simulink model "FoilSimulation23a"  (R2023a)
settings: Solver=VariableStepAuto  StartTime=0.0  StopTime=TF  RelTol=1e-3
values from neighbouring files (symbols this model uses):
  U = 0    [init.m]
  x0 = [5 ... (first row only)    [init.m]
undefined symbols (not defined in the file or in its folder): hydrofoil_model
settings Model: Creator=alank  LastModifiedBy=alank
settings RTWCC: GPUComputeCapability=5.0

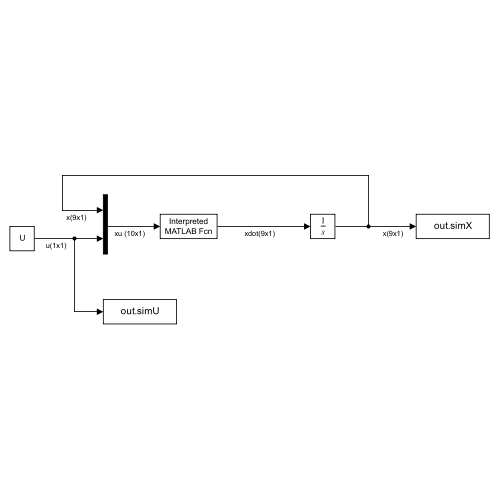
[thumbnail: Simulink's stored preview of the top-level diagram]
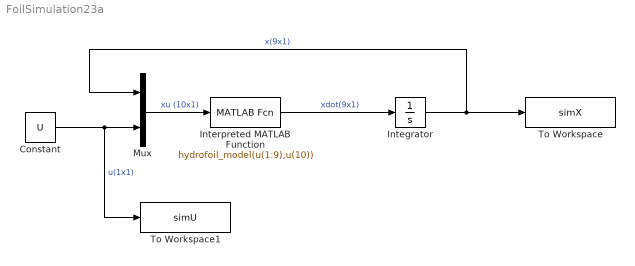
== system FoilSimulation23a ==
  Constant : Constant  Value=U
  Integrator : Integrator  InitialCondition=x0
  Interpreted MATLAB Function : MATLABFcn  MATLABFcn=hydrofoil_model(u(1:9),u(10))
  Mux : Mux  Inputs=2
  To Workspace : ToWorkspace  VariableName=simX  SaveFormat=Timeseries  SampleTime=-1
  To Workspace1 : ToWorkspace  VariableName=simU  SaveFormat=Timeseries  SampleTime=-1
  wires:
  Interpreted MATLAB Function/1 -> Integrator/1  "xdot(9x1)"
  Integrator/1 -> Mux/1, To Workspace/1  "x(9x1)"
  Constant/1 -> To Workspace1/1, Mux/2  "u(1x1)"
  Mux/1 -> Interpreted MATLAB Function/1  "xu (10x1)"
